simulink model "Flipper"  (Simulink 8.7)
settings: Solver=ode45  StartTime=0.0  StopTime=200  RelTol=1e-3
libraries: vrlib x2
settings Model: Creator=Bjoern  LastModifiedBy=birger
settings DataIOCC: SignalLoggingSaveFormat=ModelDataLogs
settings OptimizationCC: ExpressionDepthLimit=2147483647
settings DebuggingCC: SolverPrmCheckMsg=warning  FcnCallInpInsideContextMsg=UseLocalSettings  StateNameClashWarn=warning
settings SFSimCC: SimParseCustomCode=off
settings GRTTargetCC: CombineOutputUpdateFcns=off  GRTInterface=on
settings ConfigComp: CovSFcnEnable=off

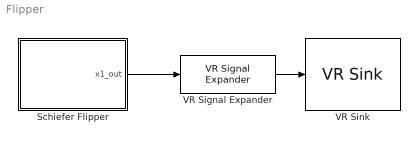
== system Flipper ==
  Schiefer Flipper : Stateflow chart  TreatAsAtomicUnit=on
  VR Signal Expander : vrlib/VR Signal Expander  outwidth=3  outidx=[1 2]
  VR Sink : vrlib/VR Sink  InstantiateOnLoad=on  SampleTime=0.05  ViewEnable=on  RemoteChange=off  RemoteView=off  FieldsWritten=Ball.translation.3.1.1.double  WorldFileName=Table.wrl  AutoView=on  VideoDimensions=[]  AllowVariableSize=off  FigureProperties="{'Position', 'Name', 'Viewpoint', 'CameraBound', 'CameraDirection', 'CameraPosition', 'CameraUpVector', 'ZoomFactor', 'Antialiasing', 'Headlight', 'Lighting', 'NavPanel', 'Sound', 'StatusBar', 'Stereo3D', 'Stereo3DCameraOffset', 'Stereo3DHIT', 'ToolBar', 'Textures', 'Transparency', 'Triad', 'Wireframe', 'NavZones', 'NavMode', 'NavSpeed', 'CaptureFileFormat', 'CaptureFileName', 'Record2DCompressMethod', 'Record2DCompressQuality', 'Record2D', 'Record2DFileName', 'Record2DFPS'; [5.0000000000000000e+00   9.5000000000000000e+01   5.7600000000000000e+02   3.5000000000000000e+02], '', 'pos2', 'on', [0.0000000000000000e+00   0.0000000000000000e+00  -1.0000000000000000e+00], [0.0000000000000000e+00   0.0000000000000000e+00   0.0000000000000000e+00], [0.0000000000000000e+00   1.0000000000000000e+00   0.0000000000000000e+00], [1.0000000000000000e+00], 'on', 'on', 'on', 'halfbar', 'on', 'on', 'off', [1.0000000149011612e-01], [0.0000000000000000e+00], 'on', 'on', 'on', 'none', 'off', 'off', 'fly', 'normal', 'tif', '%f_anim_%n.tif', 'auto', [7.5000000000000000e+01], 'off', '%f_anim_%n.avi', 'auto'}"
  wires:
  Schiefer Flipper/1(x1_out) -> VR Signal Expander/1
  VR Signal Expander/1 -> VR Sink/1

== stateflow chart Schiefer Flipper ==
  settings: updateMethod=CONTINUOUS
  state Flipper
    during:
    [v1_dot[0][0], v1_dot[1][0]]=Acc();
    x1_dot = v1;
    //output
    x1_out = x1;
  (default) -> Flipper : {Init();}
  Flipper -> Flipper [order 1] : [Wand1Kontakt()]
      | {Wand1Refl();}
  Flipper -> Flipper [order 3] : [Wand3Kontakt()]
      | {Wand3Refl();}
  Flipper -> Flipper [order 2] : [Wand2Kontakt()]
      | {Wand2Refl();}
  Flipper -> Flipper [order 4] : [HndKontakt()]
      | {HndRefl();}
  data: ax function_output double; ay function_output double; kontakt function_output boolean; kontakt function_output boolean; kontakt function_output boolean; kontakt function_output boolean; R constant double =0.25; RHnd constant double =0.8; Hnd local double size=2,1; n1 local double size=2,1; n2 local double size=2,1; n3 local double size=2,1; p1 local double size=2,1; p2 local double size=2,1; p3 local double size=2,1; t1 local double size=2,1; t2 local double size=2,1; t3 local double size=2,1; v1 local double size=2,1; x1 local double size=2,1; x1_out output double size=2,1
  data R settings: description=Radius der Kugel
  data RHnd settings: description=Radius des Zylinderhindernisses
  data Hnd settings: description=Ort des Zylinderhindernisses
  data v1 settings: updateMethod=SF_CONTINUOUS_TIME_DATA
  data x1 settings: updateMethod=SF_CONTINUOUS_TIME_DATA
  function Init:
    | function Init
    | 
    | % Hindernis und Pfosten fuer Waende
    | Hnd = [6;2.5];
    | p1 = [0;5];
    | p2 = [5;0];
    | p3 = [9;0];
    | p4 = [10;7];
    | 
    | % Kugel
    | x1 = [4;5];
    | v1 = [0;0];
    | 
    | % Normale und Tangentiale der Waende
    | t1 = (p2-p1) / norm(p2-p1);
    | n1 = [-t1(2,1); t1(1,1)];
    | t2 = (p3-p2) / norm(p3-p2);
    | n2 = [-t2(2,1) ; t2(1,1)];
    | t3 = (p4-p3) / norm(p4-p3);
    | n3 = [-t3(2,1) ; t3(1,1)];
  function [ax,ay] = Acc:
    | function [ax,ay] = Acc
    | ax = 0;
    | ay = -1;
  function kontakt = Wand1Kontakt:
    | function kontakt = Wand1Kontakt
    | kontakt = (((x1-p1)' * n1) <= R);
  function kontakt = Wand2Kontakt:
    | function kontakt = Wand2Kontakt
    | kontakt = ((x1-p2)' * n2) <= R;
  function Wand1Refl:
    | function Wand1Refl()
    | 
    | vt = v1' * t1;
    | vn = v1' * n1;
    | 
    | % Reflektierte Geschwindigkeit (mit Vektorisierung der Geschwindigkeit)
    | v1 = vt*t1 + (-vn*n1);
  function kontakt = Wand3Kontakt:
    | function kontakt = Wand3Kontakt
    | kontakt = ((x1-p3)' * n3) <= R;
  function Wand2Refl:
    | function Wand2Refl()
    | 
    | vt = v1' * t2;
    | vn = v1' * n2;
    | 
    | % Reflektierte Geschwindigkeit (mit Vektorisierung der Geschwindigkeit)
    | v1 = vt*t2 + (-vn*n2);
  function Wand3Refl:
    | function Wand3Refl()
    | 
    | vt = v1' * t3;
    | vn = v1' * n3;
    | 
    | % Reflektierte Geschwindigkeit (mit Vektorisierung der Geschwindigkeit)
    | v1 = vt*t3 + (-vn*n3);
  function kontakt = HndKontakt:
    | function kontakt = HndKontakt
    | kontakt = norm(x1 - Hnd) <= RHnd + R;
  function HndRefl:
    | function HndRefl()
    | 
    | n = (x1 - Hnd)/norm(x1- Hnd);
    | t = [n(2,1);-n(1,1)];
    | 
    | % Reflexion
    | vt = v1' * t;
    | vn = v1' * n;
    | v1 = vt*t + (-vn*n);                % Reflektierte Geschwindigkeit
